simulink model "Reas_Graph"  (R2025a)
settings: Solver=FixedStepAuto  StartTime=0.0  StopTime=inf  FixedStep=0.0005  RelTol=1e-3
values from neighbouring files (symbols this model uses):
  n = numel(files)    [LAB3_Batch_Analysis.m]
undefined symbols (not defined in the file or in its folder): Blocking, Non
libraries: amg_usbconverter_n_connect_lib x3, waijung_addon_module x1
settings Model: Creator=ACER  LastModifiedBy=ACER

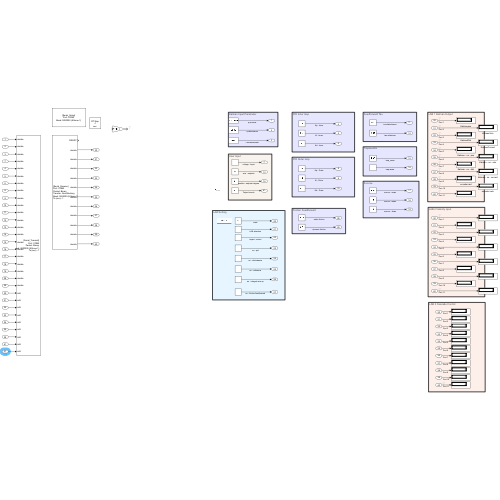
[thumbnail: Simulink's stored preview of the top-level diagram]
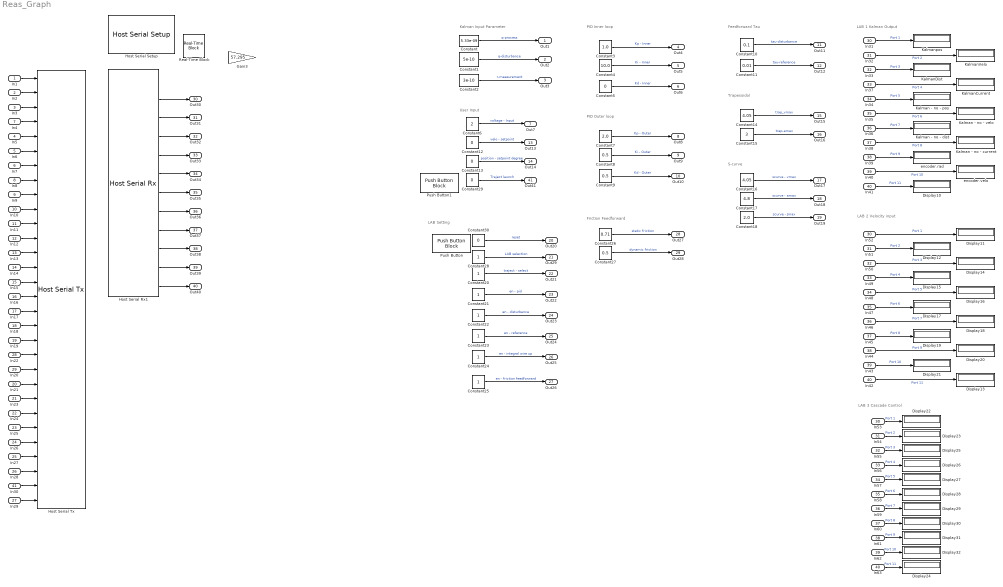
== system Reas_Graph ==
  note: User Input
  note: PID Inner loop
  note: PID Outer loop
  note: Feedforward Tau
  note: Kalman Input Parameter
  note: Trapesoidol
  note: S-curve
  note: LAB Setting
  note: Friction Feedforward
  note: LAB 1 Kalman Output
  note: LAB 2 Velocity input
  note: LAB 3 Cascade Control
  In1 : Inport
  In2 : Inport  Port=2
  In3 : Inport  Port=3
  In5 : Inport  Port=4
  In6 : Inport  Port=5
  In7 : Inport  Port=6
  In4 : Inport  Port=7
  In8 : Inport  Port=8
  In9 : Inport  Port=9
  In10 : Inport  Port=10
  In11 : Inport  Port=11
  In12 : Inport  Port=12
  In13 : Inport  Port=13
  In14 : Inport  Port=14
  In15 : Inport  Port=15
  In16 : Inport  Port=16
  In17 : Inport  Port=17
  In18 : Inport  Port=18
  In19 : Inport  Port=19
  In21 : Inport  Port=20
  In23 : Inport  Port=21
  In24 : Inport  Port=22
  In25 : Inport  Port=23
  In26 : Inport  Port=24
  In27 : Inport  Port=25
  In28 : Inport  Port=26
  In29 : Inport  Port=27
  In22 : Inport  Port=28
  In20 : Inport  Port=29
  In31 : Inport  Port=30
  In32 : Inport  Port=31
  In33 : Inport  Port=32
  In37 : Inport  Port=33
  In34 : Inport  Port=34
  In35 : Inport  Port=35
  In36 : Inport  Port=36
  In38 : Inport  Port=37
  In39 : Inport  Port=38
  In40 : Inport  Port=39
  In41 : Inport  Port=40
  In30 : Inport  Port=41
  Constant : Constant  Value=5.33e-09
  Constant1 : Constant  Value=5e-10
  Constant10 : Constant  Value=0.1
  Constant11 : Constant  Value=0.01
  Constant{5,12..13,29..30} (5 alike) : Constant  Value=0
  Constant14 : Constant  Value=4.05
  Constant15 : Constant  Value=3
  Constant16 : Constant  Value=4.05
  Constant17 : Constant  Value=4.8
  Constant18 : Constant  Value=2.0
  Constant2 : Constant  Value=3e-10
  Constant{20..25,28} (7 alike) : Constant
  Constant26 : Constant  Value=0.71
  Constant27 : Constant  Value=0.5
  Constant3 : Constant  Value=1.0
  Constant4 : Constant  Value=10.0
  Constant6 : Constant  Value=2
  Constant7 : Constant  Value=2.0
  Constant8 : Constant  Value=0.5
  Constant9 : Constant  Value=0.5
  Display{10..32} (23 alike) : Display
  Gain3 : Gain  Gain=57.295
  Host Serial Rx1 : amg_usbconverter_n_connect_lib/Host Serial Rx  conf=rx  port=<auto>  baudrate=5000000  databits=8  parity=None  stopbit=1  flowcontrol=None  transfer=Non-Blocking  timeout=5  packetmode=Binary  enableinitialvalues=off  initialvalues=[]  binheader='FF'  binterminator='0F'  porttype_double=11  porttype_single=0  porttype_int8=0  porttype_uint8=0  porttype_int16=0  porttype_uint16=0  porttype_int32=0  porttype_uint32=0  asciiformat='%d,%f'  rx_asciiterminator="CRLF (0x0D 0x0A - \"\\r\\n\")"  tx_asciiterminator="CRLF (0x0D 0x0A - \"\\r\\n\")"  sampletime=0.0005  enablecustomportlabel=off  cinputportlabel=0  coutputportlabel=A  portpinstr=0  blockid=HostSerialRx1  inputporttype=[]  inputportwidth=[]  inputportlabel={}  outputporttype=[3 0 0 0 0 0 0 0 0 0 0 0]  outputportwidth=[1 1 1 1 1 1 1 1 1 1 1 1]  outputportlabel={'READY','double','double','double','double','double','double','double','double','double','double','double'}  compat=0  optionstring=[]  autoport='COM5'
  Host Serial Setup : amg_usbconverter_n_connect_lib/Host Serial Setup  conf=setup  port=<auto>  baudrate=5000000  databits=8  parity=None  stopbit=1  flowcontrol=None  transfer=Blocking  timeout=2  packetmode=Binary  initialvalues=[]  binheader='7E 7E'  binterminator='03 03'  porttype_double=0  porttype_single=1  porttype_int8=0  porttype_uint8=0  porttype_int16=0  porttype_uint16=0  porttype_int32=0  porttype_uint32=2  asciiformat='%d %u %x'  rx_asciiterminator="CRLF (0x0D 0x0A - \"\\r\\n\")"  tx_asciiterminator="CRLF (0x0D 0x0A - \"\\r\\n\")"  sampletime=-1  enablecustomportlabel=off  cinputportlabel=0  coutputportlabel=A  portpinstr=0  blockid=HostSerialSetup  inputporttype=[]  inputportwidth=[]  inputportlabel={}  outputporttype=[]  outputportwidth=[]  outputportlabel={}  compat=0  optionstring=[]  autoport='COM5'
  Host Serial Tx : amg_usbconverter_n_connect_lib/Host Serial Tx  conf=tx  port=<auto>  baudrate=5000000  databits=8  parity=None  stopbit=1  flowcontrol=None  transfer=Blocking  timeout=2  packetmode=Binary  initialvalues=[]  binheader='FF'  binterminator='0F'  porttype_double=21  porttype_single=0  porttype_int8=9  porttype_uint8=0  porttype_int16=0  porttype_uint16=0  porttype_int32=0  porttype_uint32=0  asciiformat='%d,%f'  rx_asciiterminator="CRLF (0x0D 0x0A - \"\\r\\n\")"  tx_asciiterminator="CRLF (0x0D 0x0A - \"\\r\\n\")"  sampletime=-1  enablecustomportlabel=off  cinputportlabel=0  coutputportlabel=A  portpinstr=0  blockid=HostSerialTx  inputporttype=[0 0 0 0 0 0 0 0 0 0 0 0 0 0 0 0 0 0 0 0 0 2 2 2 2 2 2 2 2 2]  inputportwidth=[1 1 1 1 1 1 1 1 1 1 1 1 1 1 1 1 1 1 1 1 1 1 1 1 1 1 1 1 1 1]  inputportlabel={'double','double','double','double','double','double','double','double','double','double','double','double','double','double','double','double','double','double','double','double','double','int8','int8','int8','int8','int8','int8','int8','int8','int8'}  outputporttype=[]  outputportwidth=[]  outputportlabel={}  compat=0  optionstring=[]  autoport='COM5'
      settings: SourceProductName=aMG USB Converter N
  In42 : InportShadow  Port=40
  In43 : InportShadow  Port=39
  In44 : InportShadow  Port=38
  In45 : InportShadow  Port=37
  In46 : InportShadow  Port=36
  In47 : InportShadow  Port=35
  In48 : InportShadow  Port=34
  In49 : InportShadow  Port=33
  In50 : InportShadow  Port=32
  In51 : InportShadow  Port=31
  In52 : InportShadow  Port=30
  In53 : InportShadow  Port=30
  In54 : InportShadow  Port=31
  In55 : InportShadow  Port=32
  In56 : InportShadow  Port=33
  In57 : InportShadow  Port=34
  In58 : InportShadow  Port=35
  In59 : InportShadow  Port=36
  In60 : InportShadow  Port=37
  In61 : InportShadow  Port=38
  In62 : InportShadow  Port=39
  In63 : InportShadow  Port=40
  Kalman - no - current : Display
  Kalman - no - dist : Display
  Kalman - no - pos : Display
  Kalman - no - velo : Display
  KalmanCurrent : Display
  KalmanDist : Display
  KalmanVelo : Display
  Kalmanpos : Display
  Push Button : PushButtonBlock  IconOnColor=[0.0, 0.39215686274509803, 0.0]  IconOffColor=[0.0, 1.0, 0.0]  OffValue=0.000000
  Push Button1 : PushButtonBlock  IconOnColor=[0.0, 0.39215686274509803, 0.0]  IconOffColor=[0.0, 1.0, 0.0]  OffValue=0.000000
  Real-Time Block : waijung_addon_module/Real-Time Block  Priority=0  setting=Default  sampletime=-1
      settings: SourceProductName=Misc
  encoder.rad : Display
  encoder.velo : Display
  Out1 : Outport
  Out2 : Outport  Port=2
  Out3 : Outport  Port=3
  Out4 : Outport  Port=4
  Out5 : Outport  Port=5
  Out6 : Outport  Port=6
  Out7 : Outport  Port=7
  Out8 : Outport  Port=8
  Out9 : Outport  Port=9
  Out10 : Outport  Port=10
  Out11 : Outport  Port=11
  Out12 : Outport  Port=12
  Out13 : Outport  Port=13
  Out14 : Outport  Port=14
  Out15 : Outport  Port=15
  Out16 : Outport  Port=16
  Out17 : Outport  Port=17
  Out18 : Outport  Port=18
  Out19 : Outport  Port=19
  Out20 : Outport  Port=20
  Out29 : Outport  Port=21
  Out21 : Outport  Port=22
  Out22 : Outport  Port=23
  Out23 : Outport  Port=24
  Out24 : Outport  Port=25
  Out25 : Outport  Port=26
  Out26 : Outport  Port=27
  Out27 : Outport  Port=28
  Out28 : Outport  Port=29
  Out30 : Outport  Port=30
  Out31 : Outport  Port=31
  Out32 : Outport  Port=32
  Out33 : Outport  Port=33
  Out34 : Outport  Port=34
  Out35 : Outport  Port=35
  Out36 : Outport  Port=36
  Out37 : Outport  Port=37
  Out38 : Outport  Port=38
  Out39 : Outport  Port=39
  Out40 : Outport  Port=40
  Out41 : Outport  Port=41
  wires:
  Constant/1 -> Out1/1  "q-process"
  Constant1/1 -> Out2/1  "q-disturbance"
  Constant2/1 -> Out3/1  "r-measurement"
  In3/1 -> Host Serial Tx/3
  In2/1 -> Host Serial Tx/2
  In1/1 -> Host Serial Tx/1
  Constant5/1 -> Out6/1  "Kd - Inner"
  Constant3/1 -> Out4/1  "Kp - Inner"
  Constant4/1 -> Out5/1  "Ki - Inner"
  Constant6/1 -> Out7/1  "voltage - Input"
  In4/1 -> Host Serial Tx/4
  Constant7/1 -> Out8/1  "Kp - Outer"
  Constant9/1 -> Out10/1  "Kd - Outer"
  Constant8/1 -> Out9/1  "Ki - Outer"
  Constant10/1 -> Out11/1  "tau-disturbance"
  Constant11/1 -> Out12/1  "tau-reference"
  Constant12/1 -> Out13/1  "velo - setpoint"
  Constant13/1 -> Out14/1  "position - setpoint degree"
  Constant14/1 -> Out15/1  "trap_vmax"
  Constant15/1 -> Out16/1  "trap-amax"
  Constant17/1 -> Out18/1  "scurve - amax"
  Constant16/1 -> Out17/1  "scurve - vmax"
  Constant18/1 -> Out19/1  "scurve - Jmax"
  Constant20/1 -> Out21/1  "traject - select"
  Constant30/1 -> Out20/1  "reset"
  Constant21/1 -> Out22/1  "en - pid"
  Constant22/1 -> Out23/1  "en - disturbance"
  Constant23/1 -> Out24/1  "en - reference"
  Constant24/1 -> Out25/1  "en - integral wire up"
  Constant25/1 -> Out26/1  "en - friction feedforward"
  In5/1 -> Host Serial Tx/5
  In6/1 -> Host Serial Tx/6
  In7/1 -> Host Serial Tx/7
  In8/1 -> Host Serial Tx/8
  In15/1 -> Host Serial Tx/15
  In16/1 -> Host Serial Tx/16
  In13/1 -> Host Serial Tx/13
  In12/1 -> Host Serial Tx/12
  In14/1 -> Host Serial Tx/14
  In11/1 -> Host Serial Tx/11
  In10/1 -> Host Serial Tx/10
  In9/1 -> Host Serial Tx/9
  In19/1 -> Host Serial Tx/19
  In17/1 -> Host Serial Tx/17
  In21/1 -> Host Serial Tx/22
  In18/1 -> Host Serial Tx/18
  In22/1 -> Host Serial Tx/20
  In23/1 -> Host Serial Tx/23
  In20/1 -> Host Serial Tx/21
  In24/1 -> Host Serial Tx/24
  In25/1 -> Host Serial Tx/25
  Constant26/1 -> Out27/1  "static friction"
  Constant27/1 -> Out28/1  "dynamic friction"
  Constant28/1 -> Out29/1  "LAB selection"
  In29/1 -> Host Serial Tx/30
  In28/1 -> Host Serial Tx/28
  In27/1 -> Host Serial Tx/27
  In26/1 -> Host Serial Tx/26
  Host Serial Rx1/2 -> Out30/1
  Host Serial Rx1/3 -> Out31/1
  Host Serial Rx1/5 -> Out33/1
  Host Serial Rx1/4 -> Out32/1
  Host Serial Rx1/7 -> Out35/1
  Host Serial Rx1/9 -> Out37/1
  Host Serial Rx1/8 -> Out36/1
  Host Serial Rx1/6 -> Out34/1
  Host Serial Rx1/11 -> Out39/1
  Host Serial Rx1/12 -> Out40/1
  Host Serial Rx1/10 -> Out38/1
  In30/1 -> Host Serial Tx/29
  Constant29/1 -> Out41/1  "Traject launch"
  In31/1 -> Kalmanpos/1  "Port 1"
  In32/1 -> KalmanVelo/1  "Port 2"
  In33/1 -> KalmanDist/1  "Port 3"
  In37/1 -> KalmanCurrent/1  "Port 4"
  In34/1 -> Kalman - no - pos/1  "Port 5"
  In35/1 -> Kalman - no - velo/1  "Port 6"
  In36/1 -> Kalman - no - dist/1  "Port 7"
  In38/1 -> Kalman - no - current/1  "Port 8"
  In39/1 -> encoder.rad/1  "Port 9"
  In40/1 -> encoder.velo/1  "Port 10"
  In41/1 -> Display10/1  "Port 11"
  In49/1 -> Display15/1  "Port 4"
  In47/1 -> Display17/1  "Port 6"
  In48/1 -> Display16/1  "Port 5"
  In46/1 -> Display18/1  "Port 7"
  In45/1 -> Display19/1  "Port 8"
  In52/1 -> Display11/1  "Port 1"
  In51/1 -> Display12/1  "Port 2"
  In42/1 -> Display13/1  "Port 11"
  In44/1 -> Display20/1  "Port 9"
  In43/1 -> Display21/1  "Port 10"
  In50/1 -> Display14/1  "Port 3"
  In59/1 -> Display29/1  "Port 7"
  In57/1 -> Display27/1  "Port 5"
  In54/1 -> Display23/1  "Port 2"
  In61/1 -> Display31/1  "Port 9"
  In60/1 -> Display30/1  "Port 8"
  In58/1 -> Display28/1  "Port 6"
  In63/1 -> Display24/1  "Port 11"
  In56/1 -> Display26/1  "Port 4"
  In53/1 -> Display22/1  "Port 1"
  In55/1 -> Display25/1  "Port 3"
  In62/1 -> Display32/1  "Port 10"
